simulink model "Roomba_StateLinear_Cartesian"  (R2022b)
settings: Solver=FixedStepAuto  StartTime=0.0  StopTime=inf  FixedStep=0.02  RelTol=1e-3
undefined symbols (not defined in the file): offset_x, offset_y, theta_des, unicycle, X, x_des, x_f, Y, y_des, y_f
libraries: robotlib x3, dspsigops x2, simulink_extras x2
settings Model: Creator=Musta  LastModifiedBy=mustacchim
settings OptimizationCC: EnhancedBackFolding=on  PassReuseOutputArgsAs=Individual arguments  ZeroExternalMemoryAtStartup=off  ZeroInternalMemoryAtStartup=off  MaxStackSize=64  OptimizeBlockOrder=speed  DifferentSizesBufferReuse=on  OptimizationCustomize=off  EfficientTunableParamExpr=on
settings DebuggingCC: ParameterTunabilityLossMsg=error
settings HardwareCC: ProdBitPerPointer=32  ProdBitPerSizeT=32  ProdBitPerPtrDiffT=32  ProdLargestAtomicFloat=None  ProdIntDivRoundTo=Undefined  ProdEndianess=Unspecified  ProdWordSize=32  ProdHWDeviceType=Generic->Unspecified (assume 32-bit Generic)
settings SFSimCC: MATLABDynamicMemAlloc=off
settings RTWCC: Description=Embedded Coder  SystemTargetFile=ert.tlc  HardwareBoard=Robot Operating System (ROS)  TLCOptions="-aInlineSetEventsForThisBaseRateFcn=TLC_FALSE -aSuppressMultiTaskScheduler=TLC_FALSE  -aRateBasedStepFcn=0"  TemplateMakefile=ert_default_tmf  Toolchain=Catkin  TargetLang=C++
settings CodeAppCC: ForceParamTrailComments=on  IgnoreCustomStorageClasses=off  OperatorAnnotations=on  SimulinkDataObjDesc=on  SFDataObjDesc=on  InsertBlockDesc=on

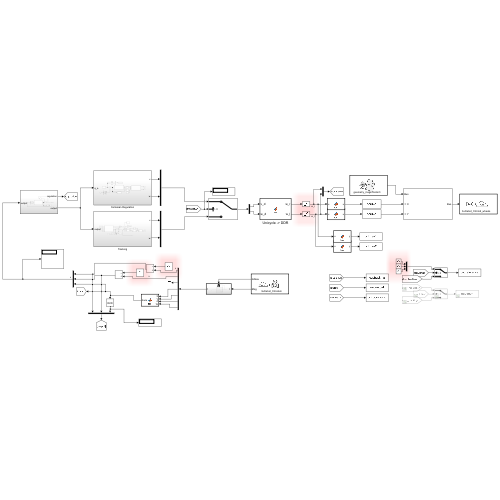
[thumbnail: Simulink's stored preview of the top-level diagram]
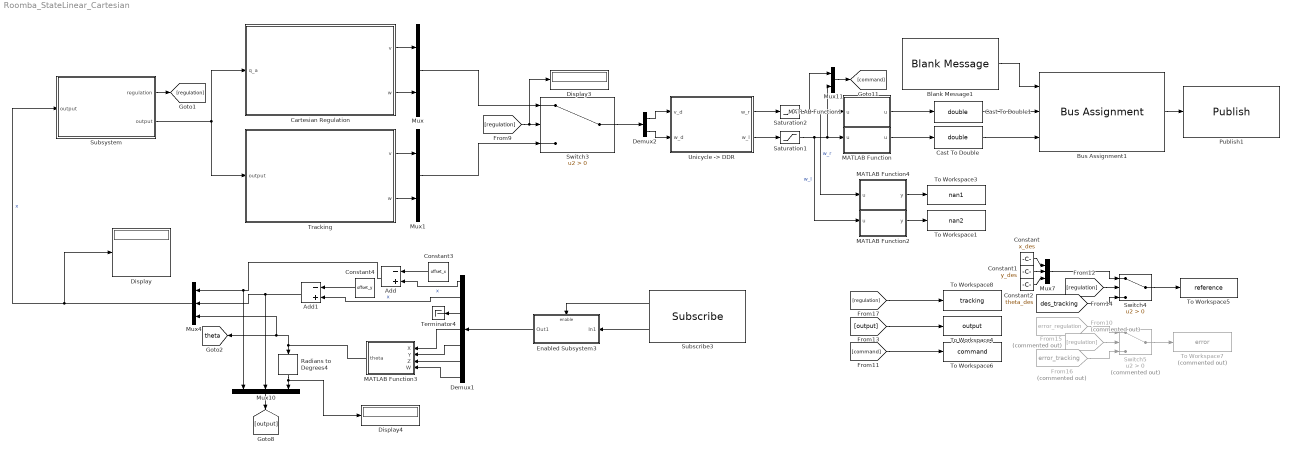
== system Roomba_StateLinear_Cartesian ==
  Add : Sum  Inputs=-+
  Add1 : Sum  Inputs=-+
  Blank Message1 : robotlib/Blank Message  messageClass=Message  entityType=geometry_msgs/Vector3  messageType=geometry_msgs/Vector3  SampleTime=0.02  legacyBusStruct=off
      settings: LibrarySourceBlock=roslib/ROS/Blank Message
  Bus Assignment1 : BusAssignment  AssignedSignals=X,Y
  Cartesian Regulation : Subsystem
  Cast To Double : DataTypeConversion  OutDataTypeStr=double  SaturateOnIntegerOverflow=off  RndMeth=Floor
  Cast To Double1 : DataTypeConversion  OutDataTypeStr=double  SaturateOnIntegerOverflow=off  RndMeth=Floor
  Constant : Constant  Value=x_des
  Constant1 : Constant  Value=y_des
  Constant2 : Constant  Value=theta_des
  Constant3 : Constant  Value=offset_x
  Constant4 : Constant  Value=offset_y
  Demux1 : Demux  Outputs=7
  Demux2 : Demux  Outputs=2
  Display : Display
  Display3 : Display
  Display4 : Display
  Enabled Subsystem3 : Subsystem  TreatAsAtomicUnit=on
  From10 : From  Commented=on  GotoTag=error_regulation  TagVisibility=global
  From15 : From  Commented=on  GotoTag=regulation
  From16 : From  Commented=on  GotoTag=error_tracking  TagVisibility=global
  MATLAB Function : MATLAB Function  TreatAsAtomicUnit=on
  MATLAB Function1 : MATLAB Function  TreatAsAtomicUnit=on
  MATLAB Function2 : MATLAB Function  TreatAsAtomicUnit=on
  MATLAB Function3 : MATLAB Function  TreatAsAtomicUnit=on
  MATLAB Function4 : MATLAB Function  TreatAsAtomicUnit=on
  Mux : Mux  Inputs=2
  Mux1 : Mux  Inputs=2
  Mux10 : Mux  Inputs=3
  Mux11 : Mux  Inputs=2
  Mux4 : Mux  Inputs=3
  Mux7 : Mux  Inputs=3
  Publish1 : robotlib/Publish  topicSource=Select from ROS network  topic=/turtlebot_03/cmd_wheels  messageType=geometry_msgs/Vector3  legacyBusStruct=off  messageQueueLength=1
      settings: LibrarySourceBlock=roslib/ROS/Publish
  Radians to Degrees4 : simulink_extras/Transformations/Radians to Degrees
  Saturation1 : Saturate  UpperLimit=unicycle.omegaWheelMax  LowerLimit=unicycle.omegaWheelMin
  Saturation2 : Saturate  UpperLimit=unicycle.omegaWheelMax  LowerLimit=unicycle.omegaWheelMin
  Subscribe3 : robotlib/Subscribe  topicSource=Select from ROS network  topic=/turtlebot_03/odom  messageType=nav_msgs/Odometry  SampleTime=0.02  legacyBusStruct=off  messageQueueLength=1
      settings: LibrarySourceBlock=roslib/ROS/Subscribe
  Subsystem : Subsystem
  Switch3 : Switch  Criteria=u2 > Threshold  SaturateOnIntegerOverflow=off  InputSameDT=off
  Switch4 : Switch  Criteria=u2 > Threshold  SaturateOnIntegerOverflow=off  InputSameDT=off
  Switch5 : Switch  Commented=on  Criteria=u2 > Threshold  SaturateOnIntegerOverflow=off  InputSameDT=off
  Terminator4 : Terminator
  To Workspace1 : ToWorkspace  VariableName=nan2  SaveFormat=Structure With Time  SampleTime=-1
  To Workspace3 : ToWorkspace  VariableName=nan1  SaveFormat=Structure With Time  SampleTime=-1
  To Workspace4 : ToWorkspace  VariableName=output  SaveFormat=Structure With Time  SampleTime=-1
  To Workspace5 : ToWorkspace  VariableName=reference  SaveFormat=Structure With Time  SampleTime=-1
  To Workspace6 : ToWorkspace  VariableName=command  SaveFormat=Structure With Time  SampleTime=-1
  To Workspace7 : ToWorkspace  Commented=on  VariableName=error  SaveFormat=Structure With Time  SampleTime=-1
  To Workspace8 : ToWorkspace  VariableName=tracking  SaveFormat=Structure With Time  SampleTime=-1
  Tracking : Subsystem
  "Unicycle -> DDR" : MATLAB Function  TreatAsAtomicUnit=on
  tag scope: theta=global
  wires:
  Radians to Degrees4/1 -> Display4/1, Mux10/3
  Demux1/7 -> MATLAB Function3/4(W)
  Demux1/6 -> MATLAB Function3/3(Z)
  "Unicycle -> DDR"/1(w_r) -> Saturation2/1
  Subscribe3/2 -> Enabled Subsystem3/1(In1)
  Demux1/5 -> MATLAB Function3/2(Y)
  Mux10/1 -> [output]
  Demux1/3 -> Terminator4/1
  Saturation2/1 -> MATLAB Function4/1(u), MATLAB Function1/1("u "), Mux11/1  "w_r"
  Saturation1/1 -> MATLAB Function2/1(u), MATLAB Function/1("u "), Mux11/2  "w_l"
  Blank Message1/1 -> Bus Assignment1/1
  Bus Assignment1/1 -> Publish1/1
  Demux1/4 -> MATLAB Function3/1(X)
  Subscribe3/1 -> Enabled Subsystem3/Enable
  Mux11/1 -> [command]
  Enabled Subsystem3/1(Out1) -> Demux1/1
  [regulation] -> Switch4/2
  [regulation] -> To Workspace8/1
  Switch5/1 -> To Workspace7/1
  Constant1/1 -> Mux7/2
  Mux7/1 -> Switch4/1
  Demux2/2 -> "Unicycle -> DDR"/2(w_d)
  [output] -> To Workspace4/1
  From10/1 -> Switch5/1
  Constant/1 -> Mux7/1
  "Unicycle -> DDR"/2(w_l) -> Saturation1/1
  From15/1 -> Switch5/2
  [des_tracking] -> Switch4/3
  Switch4/1 -> To Workspace5/1
  Demux2/1 -> "Unicycle -> DDR"/1(v_d)
  Subsystem/1(regulation) -> [regulation]
  [regulation] -> Display3/1, Switch3/2
  [command] -> To Workspace6/1
  Switch3/1 -> Demux2/1
  From16/1 -> Switch5/3
  Constant2/1 -> Mux7/3
  Mux4/1 -> Subsystem/1("output "), Display/1  "x"
  Demux1/1 -> Add/2  "x"
  Constant3/1 -> Add/1
  Constant4/1 -> Add1/1
  Demux1/2 -> Add1/2  "x"
  Add1/1 -> Mux4/2, Mux10/2
  Add/1 -> Mux4/1, Mux10/1
  Cast To Double1/1 -> Bus Assignment1/2
  Cast To Double/1 -> Bus Assignment1/3
  MATLAB Function3/1(theta) -> Mux4/3, [theta], Radians to Degrees4/1
  MATLAB Function/1(u) -> Cast To Double/1
  MATLAB Function1/1(u) -> Cast To Double1/1
  MATLAB Function2/1(y) -> To Workspace1/1
  MATLAB Function4/1(y) -> To Workspace3/1
  Cartesian Regulation/1(v) -> Mux/1
  Mux/1 -> Switch3/1
  Tracking/1(v) -> Mux1/1
  Mux1/1 -> Switch3/3
  Tracking/2(w) -> Mux1/2
  Cartesian Regulation/2(w) -> Mux/2
  Subsystem/2(output) -> Cartesian Regulation/1(q_a), Tracking/1(output)

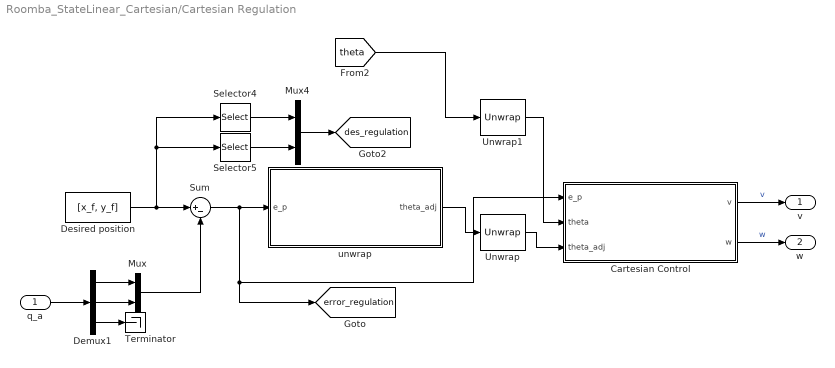
== system Roomba_StateLinear_Cartesian/Cartesian Regulation ==
  q_a : Inport
  Cartesian Control : MATLAB Function  TreatAsAtomicUnit=on
  Demux1 : Demux  Outputs=3
  Desired position : Constant  Value=[x_f, y_f]
  Mux : Mux  Inputs=2
  Mux4 : Mux  Inputs=2
  Selector4 : Selector  InputPortWidth=2  IndexOptions=Index vector (dialog)  Indices=1  OutputSizes=1
  Selector5 : Selector  InputPortWidth=2  IndexOptions=Index vector (dialog)  Indices=2  OutputSizes=1
  Sum : Sum  Inputs=|+-
  Terminator : Terminator
  Unwrap : dspsigops/Unwrap  tol=0.99*pi  InputProcessing=Columns as channels (frame based)  running=off
  Unwrap1 : dspsigops/Unwrap  tol=pi  InputProcessing=Columns as channels (frame based)  running=off
  unwrap : MATLAB Function  TreatAsAtomicUnit=on
  v : Outport
  w : Outport  Port=2
  tag scope: des_regulation=global, error_regulation=global
  wires:
  Demux1/1 -> Mux/1
  Demux1/2 -> Mux/2
  q_a/1 -> Demux1/1
  unwrap/1(theta_adj) -> Unwrap/1
  Sum/1 -> [error_regulation], Cartesian Control/1(e_p), unwrap/1(e_p)
  Mux4/1 -> [des_regulation]
  Selector5/1 -> Mux4/2
  Desired position/1 -> Selector4/1, Selector5/1, Sum/1
  Selector4/1 -> Mux4/1
  Unwrap/1 -> Cartesian Control/3(theta_adj)
  Mux/1 -> Sum/2
  Demux1/3 -> Terminator/1
  Cartesian Control/1(v) -> v/1  "v"
  Cartesian Control/2(w) -> w/1  "w"
  [theta] -> Unwrap1/1
  Unwrap1/1 -> Cartesian Control/2(theta)

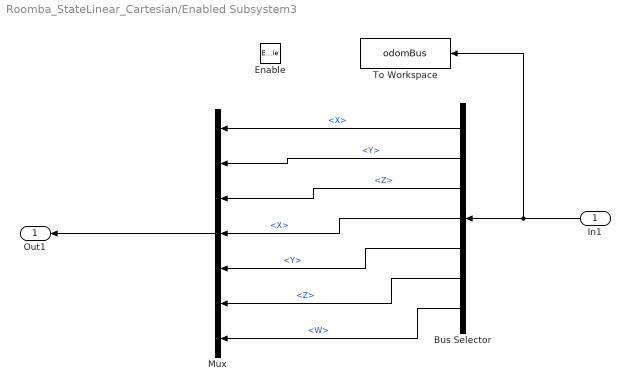
== system Roomba_StateLinear_Cartesian/Enabled Subsystem3 ==
  In1 : Inport
  Enable : EnablePort
  Bus Selector : BusSelector  OutputSignals=Pose.Pose.Position.X,Pose.Pose.Position.Y,Pose.Pose.Position.Z,Pose.Pose.Orientation.X,Pose.Pose.Orientation.Y,Pose.Pose.Orientation.Z,Pose.Pose.Orientation.W
  Mux : Mux  Inputs=7
  To Workspace : ToWorkspace  VariableName=odomBus  SaveFormat=Timeseries  SampleTime=-1
  Out1 : Outport
  wires:
  Mux/1 -> Out1/1
  Bus Selector/1 -> Mux/1  "<X>"
  Bus Selector/2 -> Mux/2  "<Y>"
  In1/1 -> To Workspace/1, Bus Selector/1
  Bus Selector/3 -> Mux/3  "<Z>"
  Bus Selector/4 -> Mux/4  "<X>"
  Bus Selector/5 -> Mux/5  "<Y>"
  Bus Selector/6 -> Mux/6  "<Z>"
  Bus Selector/7 -> Mux/7  "<W>"

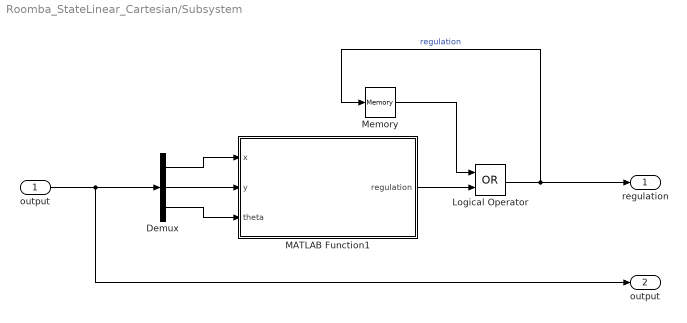
== system Roomba_StateLinear_Cartesian/Subsystem ==
  "output " : Inport
  Demux : Demux  Outputs=3
  Logical Operator : Logic  Operator=OR  AllPortsSameDT=off  OutDataTypeStr=boolean
  MATLAB Function1 : MATLAB Function  TreatAsAtomicUnit=on
  Memory : Memory
  regulation : Outport
  output : Outport  Port=2
  wires:
  Memory/1 -> Logical Operator/1
  Logical Operator/1 -> regulation/1, Memory/1  "regulation"
  MATLAB Function1/1(regulation) -> Logical Operator/2
  "output "/1 -> output/1, Demux/1
  Demux/3 -> MATLAB Function1/3(theta)
  Demux/2 -> MATLAB Function1/2(y)
  Demux/1 -> MATLAB Function1/1(x)

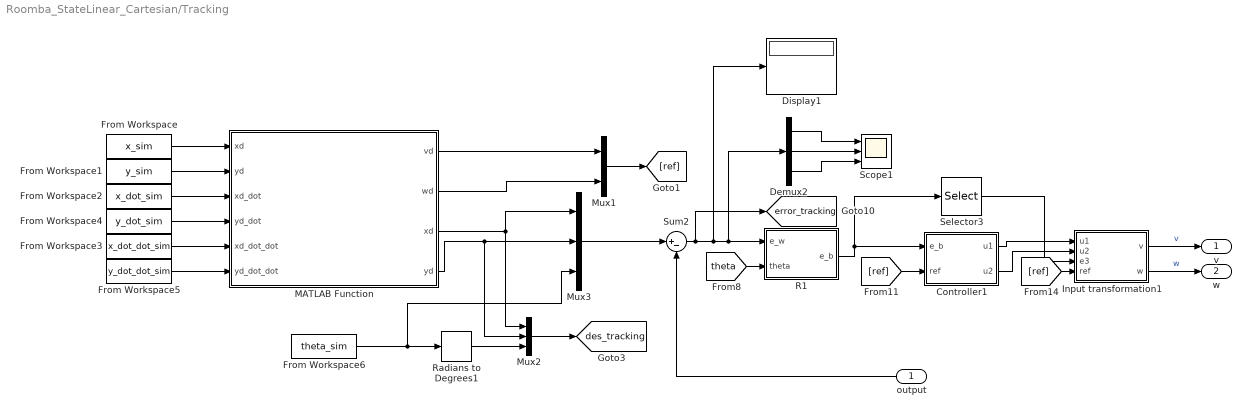
== system Roomba_StateLinear_Cartesian/Tracking ==
  output : Inport
  Controller1 : MATLAB Function  TreatAsAtomicUnit=on
  Demux2 : Demux  Outputs=3
  Display1 : Display
  From Workspace : FromWorkspace  VariableName=x_sim
  From Workspace1 : FromWorkspace  VariableName=y_sim
  From Workspace2 : FromWorkspace  VariableName=x_dot_sim
  From Workspace3 : FromWorkspace  VariableName=x_dot_dot_sim
  From Workspace4 : FromWorkspace  VariableName=y_dot_sim
  From Workspace5 : FromWorkspace  VariableName=y_dot_dot_sim
  From Workspace6 : FromWorkspace  VariableName=theta_sim
  Input transformation1 : MATLAB Function  TreatAsAtomicUnit=on
  MATLAB Function : MATLAB Function  TreatAsAtomicUnit=on
  Mux1 : Mux  Inputs=2
  Mux2 : Mux  Inputs=3
  Mux3 : Mux  Inputs=3
  R1 : MATLAB Function  TreatAsAtomicUnit=on
  Radians to Degrees1 : simulink_extras/Transformations/Radians to Degrees
  Scope1 : Scope  NumInputPorts=3
  Selector3 : Selector  InputPortWidth=3  IndexOptions=Index vector (dialog)  Indices=3  OutputSizes=1
  Sum2 : Sum  Inputs=|+-
  v : Outport
  w : Outport  Port=2
  tag scope: des_tracking=global, error_tracking=global
  wires:
  Sum2/1 -> [error_tracking], Display1/1, R1/1(e_w), Demux2/1
  [theta] -> R1/2(theta)
  Input transformation1/1(v) -> v/1  "v"
  Selector3/1 -> Input transformation1/3(e3)
  Demux2/2 -> Scope1/2
  R1/1(e_b) -> Selector3/1, Controller1/1(e_b)
  Controller1/1(u1) -> Input transformation1/1(u1)
  Demux2/1 -> Scope1/1
  [ref] -> Controller1/2(ref)
  [ref] -> Input transformation1/4(ref)
  Demux2/3 -> Scope1/3
  Controller1/2(u2) -> Input transformation1/2(u2)
  output/1 -> Sum2/2
  Input transformation1/2(w) -> w/1  "w"
  Radians to Degrees1/1 -> Mux2/3
  From Workspace5/1 -> MATLAB Function/6(yd_dot_dot)
  From Workspace1/1 -> MATLAB Function/2("yd ")
  MATLAB Function/1(vd) -> Mux1/1
  Mux1/1 -> [ref]
  From Workspace3/1 -> MATLAB Function/5(xd_dot_dot)
  MATLAB Function/3(xd) -> Mux3/1, Mux2/1
  From Workspace/1 -> MATLAB Function/1("xd ")
  MATLAB Function/2(wd) -> Mux1/2
  From Workspace4/1 -> MATLAB Function/4(yd_dot)
  MATLAB Function/4(yd) -> Mux2/2, Mux3/2
  Mux2/1 -> [des_tracking]
  From Workspace6/1 -> Radians to Degrees1/1, Mux3/3
  From Workspace2/1 -> MATLAB Function/3(xd_dot)
  Mux3/1 -> Sum2/1

== matlab function Roomba_StateLinear_Cartesian/Tracking/R1 ==
  data: e_w input; e_b output; theta input
function e_b  = fcn(e_w, theta)
    
    R = [cos(theta), sin(theta), 0;
        -sin(theta), cos(theta), 0;
         0, 0, 1];

    e_b = R * e_w;

end

== matlab function Roomba_StateLinear_Cartesian/Subsystem/MATLAB Function1 ==
  data: x input; regulation output; y input; theta input
function regulation = fcn(x,y,theta)

    x_des = 1.51;
    y_des = -0.5;

    th = 0.01;

    if (abs(x)<abs(x_des)+th) && (abs(x)>abs(x_des)-th) && (abs(y)<abs(y_des)+th) && (abs(y)>abs(y_des)-th)
        regulation = 1;
    else
        regulation = 0;
    end

end

== matlab function Roomba_StateLinear_Cartesian/Unicycle -> DDR ==
  data: v_d input; w_r output; w_d input; w_l output
function [w_r, w_l] = fcn(v_d, w_d)

    d = 0.165;
    r = 0.034;

    w_r = ((2 * v_d) + (w_d * d)) / (2 * r);
    w_l = ((2 * v_d) - (w_d * d)) / (2 * r);

end

== matlab function Roomba_StateLinear_Cartesian/Cartesian Regulation/unwrap ==
  data: theta_adj output; e_p input

function theta_adj = unwrap(e_p)

    theta_adj = atan2(e_p(2),e_p(1));

end

== matlab function Roomba_StateLinear_Cartesian/MATLAB Function3 ==
  data: X input; theta output; Y input; Z input; W input
function theta = fcn(X, Y, Z, W)

    q_x = X;
    q_y = Y;
    q_z = Z;
    q_w = W;
    
    q = cat(2,q_w,q_x,q_y,q_z); 
    eulZYX = quat2eul(q,'ZYX');
    theta = eulZYX(1);
    
end

== matlab function Roomba_StateLinear_Cartesian/MATLAB Function ==
  data: u input; u output
function u = fcn(u)


    if (isnan(u))
        u = 0.1;
    end

end

== matlab function Roomba_StateLinear_Cartesian/MATLAB Function1 ==
  data: u input; u output
function u = fcn(u)

    if (isnan(u))
        u = 0.1;
    end

end

== matlab function Roomba_StateLinear_Cartesian/MATLAB Function2 ==
  data: u input; y output
function y = fcn(u)

    y = 0;

    if (isnan(u))
        y = 1;
    end

end

== matlab function Roomba_StateLinear_Cartesian/MATLAB Function4 ==
  data: u input; y output
function y = fcn(u)

    y = 0;

    if (isnan(u))
        y = 1;
    end

end

== matlab function Roomba_StateLinear_Cartesian/Tracking/Controller1 ==
  data: e_b input; u1 output; ref input; u2 output
function [u1,u2] = fcn(e_b, ref)

    %#codegen
    coder.extrinsic('evalin')
    a = 0;                  % Needed in order to set variable class correctly
    zeta = 0;                  % Needed in order to set variable class correctly
    a = evalin('base','a'); % Read value from workspace
    zeta = evalin('base','zeta'); % Read value from workspace

    k1 = 2*zeta*a;
    k2 = (a^2 - ref(2)^2) / ref(1);
    k3 = 2*zeta*a;

    u1 = -k1*e_b(1);
    u2 = -k2*e_b(2) -k3*e_b(3);

end

== matlab function Roomba_StateLinear_Cartesian/Cartesian Regulation/Cartesian Control ==
  data: v output; w output; e_p input; theta input; theta_adj input
function [v,w] = cartesian_controller(e_p, theta, theta_adj)

    %#codegen
    coder.extrinsic('evalin')
    K_v = 0;                  % Needed in order to set variable class correctly
    K_w = 0;                  % Needed in order to set variable class correctly
    K_v = evalin('base','K_v'); % Read value from workspace
    K_w = evalin('base','K_w'); % Read value from workspace

    v = K_v * (e_p(1)*cos(theta) + e_p(2)*sin(theta));
    w = K_w * (theta_adj - theta);

%     distance = sqrt((ep(1)).^2+(ep(2)).^2);
% 
%     if distance < .1
%         v = .5*v;
%         w = .5*w;
%         if distance < .04
%             v = 0;
%             w = 0; 
%         end
%     end 

end

== matlab function Roomba_StateLinear_Cartesian/Tracking/Input transformation1 ==
  data: u1 input; v output; u2 input; e3 input; w output; ref input
function [v, w] = fcn(u1, u2, e3, ref)

    v = ref(1)*cos(e3) - u1;
    w = ref(2) - u2;

end

== matlab function Roomba_StateLinear_Cartesian/Tracking/MATLAB Function ==
  data: xd input; vd output; yd input; xd_dot input; yd_dot input; xd_dot_dot input; yd_dot_dot input; wd output; xd output; yd output
function [vd, wd, xd, yd] = fcn(xd, yd, xd_dot, yd_dot, xd_dot_dot, yd_dot_dot)
    
    vd = sqrt(xd_dot.^2 + yd_dot.^2);
    wd = (xd_dot.*yd_dot_dot - xd_dot_dot.*yd_dot) / (xd_dot.^2 + yd_dot.^2);

    xd = xd;
    yd = yd;

end
